simulink model "ModelWithSimulator"  (R2018a)
settings: Solver=ode4  StartTime=0.0  StopTime=inf  FixedStep=.001  RelTol=1e-2
undefined symbols (not defined in the file): car, initBeta, initR, initV
libraries: ephysenetlib x5, realtime_pacer_lib x1
settings Model: Creator=efrem  LastModifiedBy=efrem
settings SolverCC: AlgebraicLoopSolver=LineSearch
settings CodeAppCC: StateflowObjectComments=on

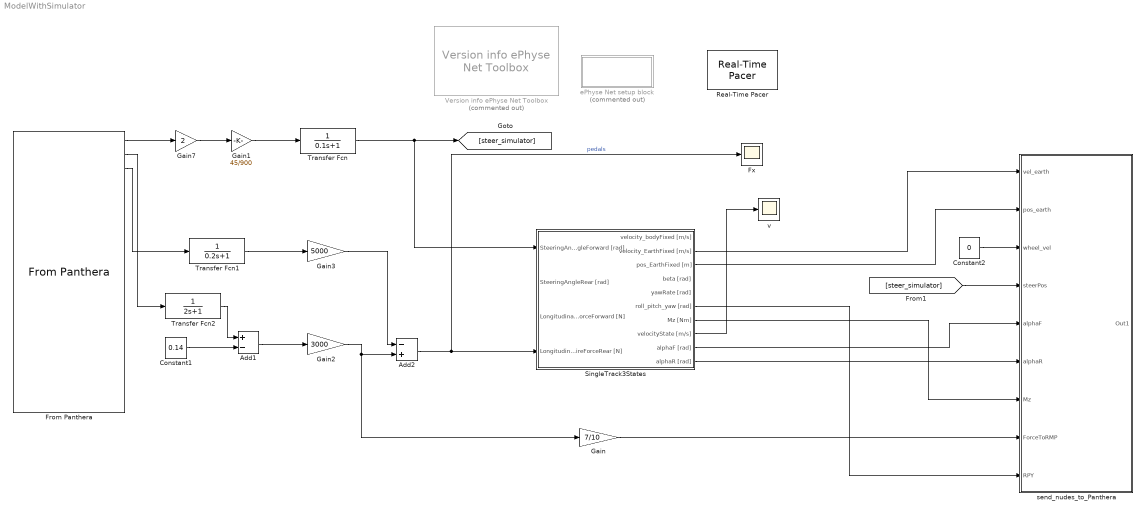
== system ModelWithSimulator ==
  Add1 : Sum  Inputs=+-
  Add2 : Sum  Inputs=-+
  Constant1 : Constant  Value=0.14
  Constant2 : Constant  Value=0
  From Panthera : ephysenetlib/Input blocks/From Panthera
  Fx : Scope
  Gain : Gain  Gain=7/10
  Gain1 : Gain  Gain=45/900
  Gain2 : Gain  Gain=3000
  Gain3 : Gain  Gain=5000
  Gain7 : Gain  Gain=2
  Real-Time Pacer : realtime_pacer_lib/Real-Time Pacer  simTimePerRealTime=1
  SingleTrack3States : Subsystem
  Transfer Fcn : TransferFcn  Denominator=[0.1 1]
  Transfer Fcn1 : TransferFcn  Denominator=[0.2 1]
  Transfer Fcn2 : TransferFcn  Denominator=[2 1]
  Version info ePhyse Net Toolbox : ephysenetlib/Setup blocks/Version info ePhyse Net Toolbox  Commented=on  InitialBlockCM=None  BlockCM=None  Frame=on  DisplayStringWithTags=|  HorizontalTextAlignment=Center  LeftAlignmentValue=0.5  SourceBlockDiagram=MODEL  TagMaxNumber=20
      | ePhyse Net Toolbox
      | Version:  1.0
      | Revision: $Rev: 1.0 $
      | 
      | © Cruden B.V., 2012
  ePhyse Net setup block : Subsystem  Commented=on  AncestorBlock=ephysenetlib/Setup blocks/Setup block
  send_nudes_to_Panthera : Subsystem
  v : Scope
  wires:
  SingleTrack3States/2(velocity_EarthFixed [m/s]) -> send_nudes_to_Panthera/1(vel_earth)
  Gain7/1 -> Gain1/1
  Gain1/1 -> Transfer Fcn/1
  SingleTrack3States/10(alphaR [rad]) -> send_nudes_to_Panthera/6(alphaR)
  Constant2/1 -> send_nudes_to_Panthera/3(wheel_vel)
  Constant1/1 -> Add1/2
  Transfer Fcn2/1 -> Add1/1
  Transfer Fcn1/1 -> Gain3/1
  From Panthera/2 -> Transfer Fcn2/1
  Add1/1 -> Gain2/1
  SingleTrack3States/9(alphaF [rad]) -> send_nudes_to_Panthera/5(alphaF)
  Add2/1 -> Fx/1, SingleTrack3States/4(LongitudinalTireForceRear [N])  "pedals"
  From Panthera/3 -> Transfer Fcn1/1
  SingleTrack3States/7(Mz [Nm]) -> send_nudes_to_Panthera/7(Mz)
  Gain2/1 -> Gain/1, Add2/2
  SingleTrack3States/3(pos_EarthFixed [m]) -> send_nudes_to_Panthera/2(pos_earth)
  Gain3/1 -> Add2/1
  SingleTrack3States/6(roll_pitch_yaw [rad]) -> send_nudes_to_Panthera/9("RPY ")
  [steer_simulator] -> send_nudes_to_Panthera/4(steerPos)
  From Panthera/1 -> Gain7/1
  Transfer Fcn/1 -> [steer_simulator], SingleTrack3States/1(SteeringAngleForward [rad])
  Gain/1 -> send_nudes_to_Panthera/8(ForceToRMP)
  SingleTrack3States/8(velocityState [m/s]) -> v/1

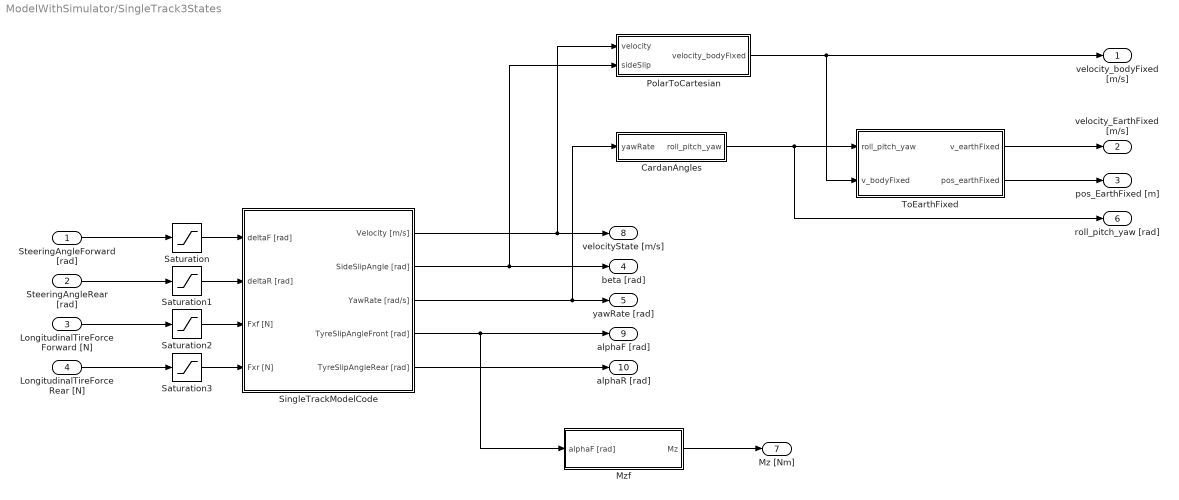
== system ModelWithSimulator/SingleTrack3States ==
  SteeringAngleForward [rad] : Inport
  SteeringAngleRear [rad] : Inport  Port=2
  LongitudinalTireForceForward [N] : Inport  Port=3
  LongitudinalTireForceRear [N] : Inport  Port=4
  CardanAngles : Subsystem
  Mzf : Subsystem
  PolarToCartesian : Subsystem
  Saturation : Saturate  UpperLimit=pi/3  LowerLimit=-pi/3  ZeroCross=off
  Saturation1 : Saturate  UpperLimit=pi/3  LowerLimit=-pi/3  ZeroCross=off
  Saturation2 : Saturate  UpperLimit=10000  LowerLimit=-10000  ZeroCross=off
  Saturation3 : Saturate  UpperLimit=10000  LowerLimit=-10000  ZeroCross=off
  SingleTrackModelCode : Subsystem
  ToEarthFixed : Subsystem
  velocity_bodyFixed [m/s] : Outport
  velocity_EarthFixed [m/s] : Outport  Port=2
  pos_EarthFixed [m] : Outport  Port=3
  beta [rad] : Outport  Port=4
  yawRate [rad] : Outport  Port=5
  roll_pitch_yaw [rad] : Outport  Port=6
  Mz [Nm] : Outport  Port=7
  velocityState [m/s] : Outport  Port=8
  alphaF [rad] : Outport  Port=9
  alphaR [rad] : Outport  Port=10
  wires:
  SingleTrackModelCode/3(YawRate [rad/s]) -> CardanAngles/1(yawRate), yawRate [rad]/1
  ToEarthFixed/2(pos_earthFixed) -> pos_EarthFixed [m]/1
  PolarToCartesian/1(velocity_bodyFixed) -> ToEarthFixed/2(v_bodyFixed), velocity_bodyFixed [m/s]/1
  SingleTrackModelCode/2(SideSlipAngle [rad]) -> PolarToCartesian/2(sideSlip), beta [rad]/1
  ToEarthFixed/1(v_earthFixed) -> velocity_EarthFixed [m/s]/1
  CardanAngles/1(roll_pitch_yaw) -> roll_pitch_yaw [rad]/1, ToEarthFixed/1(roll_pitch_yaw)
  SteeringAngleForward [rad]/1 -> Saturation/1
  LongitudinalTireForceForward [N]/1 -> Saturation2/1
  LongitudinalTireForceRear [N]/1 -> Saturation3/1
  Saturation1/1 -> SingleTrackModelCode/2(deltaR [rad])
  Saturation2/1 -> SingleTrackModelCode/3(Fxf [N])
  Saturation3/1 -> SingleTrackModelCode/4(Fxr [N])
  SteeringAngleRear [rad]/1 -> Saturation1/1
  Saturation/1 -> SingleTrackModelCode/1(deltaF [rad])
  SingleTrackModelCode/1(Velocity [m/s]) -> PolarToCartesian/1(velocity), velocityState [m/s]/1
  SingleTrackModelCode/4(TyreSlipAngleFront [rad]) -> Mzf/1(alphaF [rad]), alphaF [rad]/1
  SingleTrackModelCode/5(TyreSlipAngleRear [rad]) -> alphaR [rad]/1
  Mzf/1(Mz) -> Mz [Nm]/1

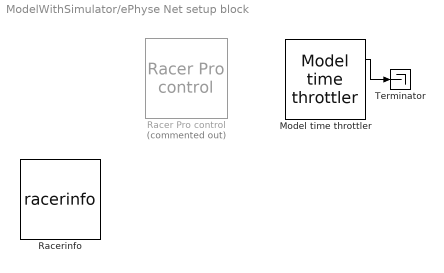
== system ModelWithSimulator/ePhyse Net setup block ==
  Model time throttler : ephysenetlib/Setup blocks/Model time throttler  enable=on
  Racer Pro control : ephysenetlib/Setup blocks/Racer Pro control  Commented=on
  Racerinfo : S-Function  Priority=5  FunctionName=racerinfo  Parameters=3  SFunctionDeploymentMode=off  EnableBusSupport=off
  Terminator : Terminator
  wires:
  Model time throttler/1 -> Terminator/1

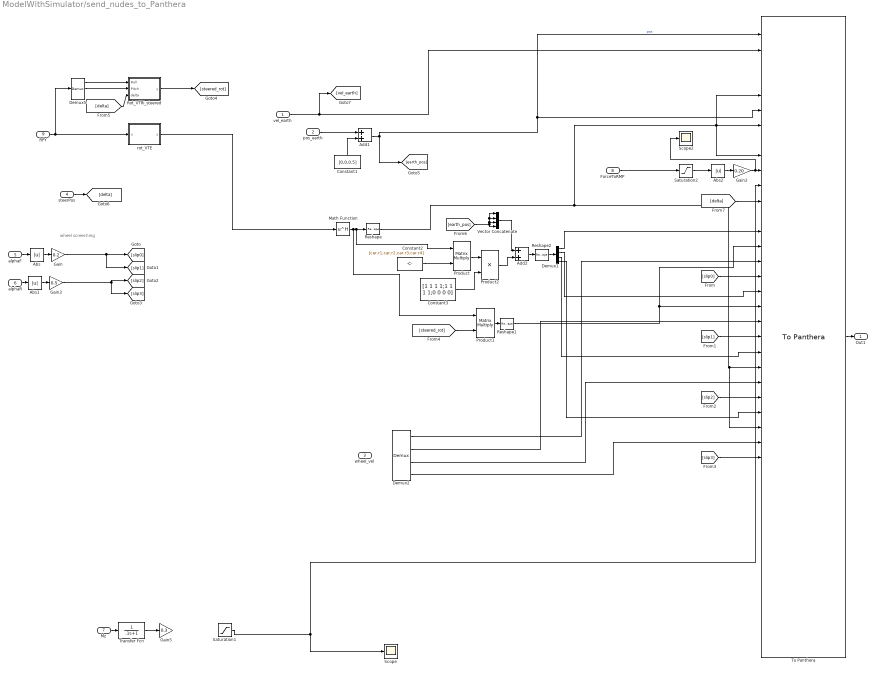
== system ModelWithSimulator/send_nudes_to_Panthera ==
  note: wheel screeching
  vel_earth : Inport
  pos_earth : Inport  Port=2
  wheel_vel : Inport  Port=3
  steerPos : Inport  Port=4
  alphaF : Inport  Port=5
  alphaR : Inport  Port=6
  Mz : Inport  Port=7
  ForceToRMP : Inport  Port=8
  "RPY " : Inport  Port=9
  Abs : Abs  ZeroCross=off
  Abs1 : Abs  ZeroCross=off
  Abs2 : Abs
  Add1 : Sum
  Add2 : Sum
  Constant1 : Constant  Value=[0,0,0.5]
  Constant2 : Constant  Value=[car.r1,car.r2,car.r3,car.r4]
  Constant3 : Constant  Value=[1 1 1 1;1 1 1 1;0 0 0 0]
  Demux1 : Demux
  Demux2 : Demux
  Demux5 : Demux  Outputs=3
  Gain : Gain  Gain=0.2
  Gain2 : Gain  Gain=0.20
  Gain3 : Gain  Gain=0.5
  Gain5 : Gain  Gain=0.3
  Math Function : Math  Operator=hermitian  SaturateOnIntegerOverflow=on
  Product : Product  Multiplication=Matrix(*)
  Product1 : Product  Multiplication=Matrix(*)
  Product2 : Product
  Reshape : Reshape
  Reshape1 : Reshape
  Reshape2 : Reshape  OutputDimensionality=Customize  OutputDimensions=[1,12]
  Rot_VTRi_steered : MATLAB Function  TreatAsAtomicUnit=on
  Saturation1 : Saturate  UpperLimit=150  LowerLimit=-150
  Saturation2 : Saturate  UpperLimit=inf  LowerLimit=0
  Scope : Scope
  Scope2 : Scope
  To Panthera : ephysenetlib/Output blocks/To Panthera
  Transfer Fcn : TransferFcn  Denominator=[.1 1]
  Vector Concatenate : Concatenate  NumInputs=4  Mode=Multidimensional array  ConcatenateDimension=2
  rot_VTE : MATLAB Function  TreatAsAtomicUnit=on
  Out1 : Outport
  wires:
  To Panthera/1 -> Out1/1
  vel_earth/1 -> [vel_earth], To Panthera/2
  rot_VTE/1(y) -> Math Function/1
  Math Function/1 -> Product1/1, Product/1, Reshape/1
  pos_earth/1 -> Add1/1
  Constant1/1 -> Add1/2
  [slip0] -> To Panthera/17
  [slip1] -> To Panthera/21
  [slip2] -> To Panthera/25
  [slip3] -> To Panthera/29
  Rot_VTRi_steered/1(y) -> [steered_rot]
  Constant2/1 -> Product/2
  Vector Concatenate/1 -> Add2/1
  [earth_pos] -> Vector Concatenate/4, Vector Concatenate/1, Vector Concatenate/2, Vector Concatenate/3
  Add2/1 -> Reshape2/1
  Reshape2/1 -> Demux1/1
  Demux1/1 -> To Panthera/14
  Demux1/2 -> To Panthera/18
  Demux1/3 -> To Panthera/22
  Demux1/4 -> To Panthera/26
  [steered_rot] -> Product1/2
  Product1/1 -> Reshape1/1
  Reshape1/1 -> To Panthera/15, To Panthera/19
  Reshape/1 -> To Panthera/9, To Panthera/5, To Panthera/7, To Panthera/27, To Panthera/23
  Add1/1 -> [earth_pos], To Panthera/6, To Panthera/1  "pos"
  Product/1 -> Product2/1
  Product2/1 -> Add2/2
  Constant3/1 -> Product2/2
  Demux2/1 -> To Panthera/16
  Demux2/2 -> To Panthera/20
  Demux2/3 -> To Panthera/24
  Demux2/4 -> To Panthera/28
  steerPos/1 -> [delta]
  alphaF/1 -> Abs/1
  Abs/1 -> Gain/1
  ForceToRMP/1 -> Saturation2/1
  Gain2/1 -> Scope2/1, To Panthera/10
  Abs2/1 -> Gain2/1
  Saturation2/1 -> Abs2/1
  "RPY "/1 -> rot_VTE/1(u), Demux5/1
  Demux5/1 -> Rot_VTRi_steered/1(Roll)
  Demux5/2 -> Rot_VTRi_steered/2(Pitch)
  [delta] -> Rot_VTRi_steered/3(delta)
  [delta] -> To Panthera/12
  Mz/1 -> Transfer Fcn/1
  Saturation1/1 -> To Panthera/11, Scope/1
  Abs1/1 -> Gain3/1
  alphaR/1 -> Abs1/1
  Gain/1 -> [slip1], [slip0]
  Gain3/1 -> [slip2], [slip3]
  Transfer Fcn/1 -> Gain5/1

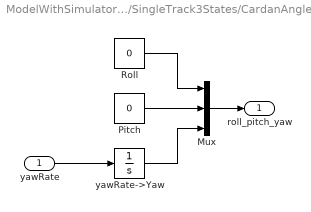
== system ModelWithSimulator/SingleTrack3States/CardanAngles ==
  yawRate : Inport
  Mux : Mux  Inputs=3
  Pitch : Constant  Value=0
  Roll : Constant  Value=0
  yawRate->Yaw : Integrator
  roll_pitch_yaw : Outport
  wires:
  Roll/1 -> Mux/1
  Mux/1 -> roll_pitch_yaw/1
  Pitch/1 -> Mux/2
  yawRate->Yaw/1 -> Mux/3
  yawRate/1 -> yawRate->Yaw/1

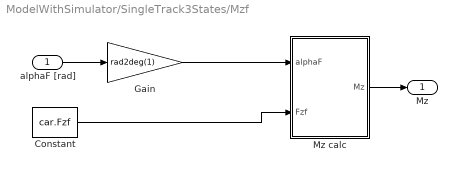
== system ModelWithSimulator/SingleTrack3States/Mzf ==
  alphaF [rad] : Inport
  Constant : Constant  Value=car.Fzf
  Gain : Gain  Gain=rad2deg(1)
  Mz calc : MATLAB Function  TreatAsAtomicUnit=on
  Mz : Outport
  wires:
  Mz calc/1(Mz) -> Mz/1
  Constant/1 -> Mz calc/2(Fzf)
  Gain/1 -> Mz calc/1(alphaF)
  alphaF [rad]/1 -> Gain/1

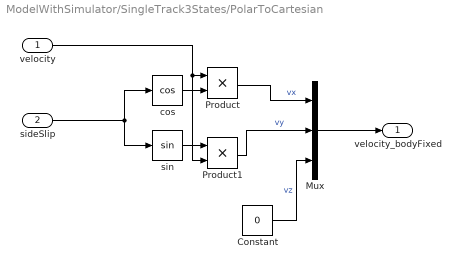
== system ModelWithSimulator/SingleTrack3States/PolarToCartesian ==
  velocity : Inport
  sideSlip : Inport  Port=2
  Constant : Constant  Value=0
  Mux : Mux  Inputs=3
  Product : Product
  Product1 : Product
  cos : Trigonometry  Operator=cos
  sin : Trigonometry
  velocity_bodyFixed : Outport
  wires:
  cos/1 -> Product/2
  sin/1 -> Product1/1
  Product/1 -> Mux/1  "vx"
  velocity/1 -> Product/1, Product1/2
  Product1/1 -> Mux/2  "vy"
  sideSlip/1 -> cos/1, sin/1
  Mux/1 -> velocity_bodyFixed/1
  Constant/1 -> Mux/3  "vz"

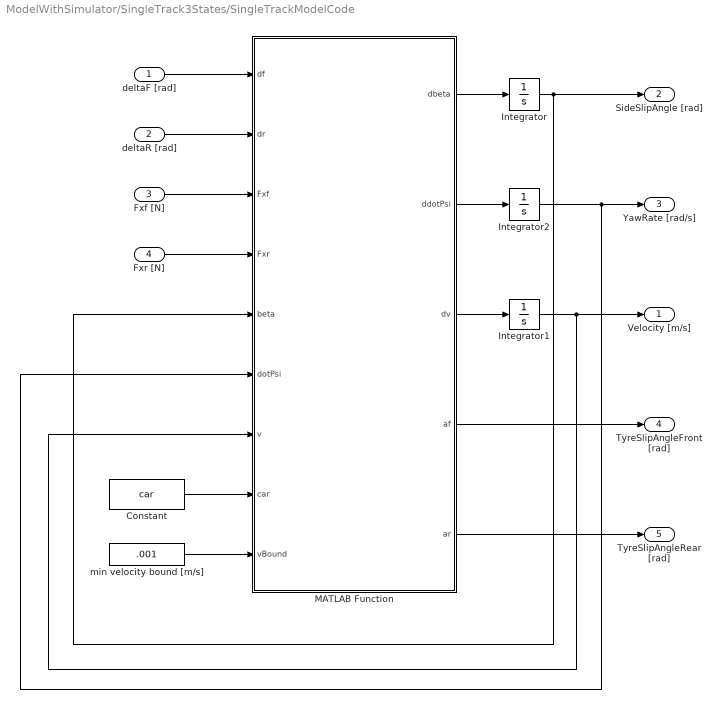
== system ModelWithSimulator/SingleTrack3States/SingleTrackModelCode ==
  deltaF [rad] : Inport
  deltaR [rad] : Inport  Port=2
  Fxf [N] : Inport  Port=3
  Fxr [N] : Inport  Port=4
  Constant : Constant  Value=car  OutDataTypeStr=Bus: car_bus
  Integrator : Integrator  InitialCondition=initBeta  UpperSaturationLimit=pi/2  LowerSaturationLimit=-pi/2  ZeroCross=off
  Integrator1 : Integrator  InitialCondition=initV  UpperSaturationLimit=100  LowerSaturationLimit=0.01  IgnoreLimit=on  ZeroCross=off
  Integrator2 : Integrator  InitialCondition=initR
  MATLAB Function : MATLAB Function  TreatAsAtomicUnit=on
  min velocity bound [m/s] : Constant  Value=.001
  Velocity [m/s] : Outport
  SideSlipAngle [rad] : Outport  Port=2
  YawRate [rad/s] : Outport  Port=3
  TyreSlipAngleFront [rad] : Outport  Port=4
  TyreSlipAngleRear [rad] : Outport  Port=5
  wires:
  MATLAB Function/1(dbeta) -> Integrator/1
  MATLAB Function/2(ddotPsi) -> Integrator2/1
  MATLAB Function/3(dv) -> Integrator1/1
  Integrator/1 -> SideSlipAngle [rad]/1, MATLAB Function/5(beta)
  Integrator2/1 -> YawRate [rad/s]/1, MATLAB Function/6(dotPsi)
  Integrator1/1 -> Velocity [m/s]/1, MATLAB Function/7(v)
  deltaF [rad]/1 -> MATLAB Function/1(df)
  deltaR [rad]/1 -> MATLAB Function/2(dr)
  Fxf [N]/1 -> MATLAB Function/3(Fxf)
  Fxr [N]/1 -> MATLAB Function/4(Fxr)
  min velocity bound [m/s]/1 -> MATLAB Function/9(vBound)
  MATLAB Function/4(af) -> TyreSlipAngleFront [rad]/1
  MATLAB Function/5(ar) -> TyreSlipAngleRear [rad]/1
  Constant/1 -> MATLAB Function/8(car)

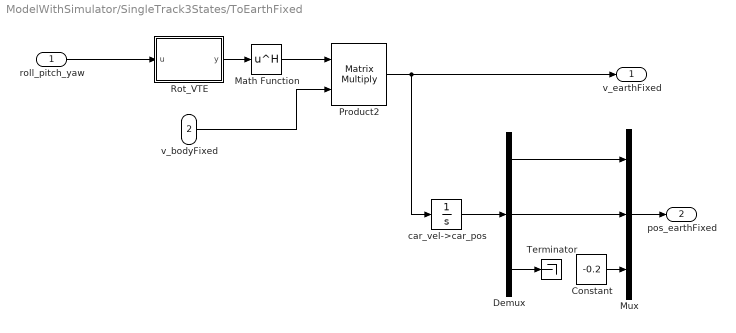
== system ModelWithSimulator/SingleTrack3States/ToEarthFixed ==
  roll_pitch_yaw : Inport
  v_bodyFixed : Inport  Port=2
  Constant : Constant  Value=-0.2
  Demux : Demux  Outputs=3
  Math Function : Math  Operator=hermitian  SaturateOnIntegerOverflow=on
  Mux : Mux  Inputs=3
  Product2 : Product  Multiplication=Matrix(*)
  Rot_VTE : MATLAB Function  TreatAsAtomicUnit=on
  Terminator : Terminator
  car_vel->car_pos : Integrator
  v_earthFixed : Outport
  pos_earthFixed : Outport  Port=2
  wires:
  Rot_VTE/1(y) -> Math Function/1
  roll_pitch_yaw/1 -> Rot_VTE/1(u)
  Constant/1 -> Mux/3
  car_vel->car_pos/1 -> Demux/1
  Product2/1 -> v_earthFixed/1, car_vel->car_pos/1
  Demux/1 -> Mux/1
  Demux/2 -> Mux/2
  v_bodyFixed/1 -> Product2/2
  Mux/1 -> pos_earthFixed/1
  Math Function/1 -> Product2/1
  Demux/3 -> Terminator/1

== matlab function ModelWithSimulator/SingleTrack3States/ToEarthFixed/Rot_VTE ==
  data: u input; y output
function y = fcn(u)
y = Rot_VTE(u);

== matlab function ModelWithSimulator/SingleTrack3States/Mzf/Mz calc ==
  data: alphaF input; Mz output; Fzf input
function Mz = fcn(alphaF, Fzf)
Bz = .15;
Cz = 2.3;
Dz = -.05 * Fzf;
Ez = -10;
Mz = Dz*sin((Cz*atan(Bz*alphaF - Ez*(Bz*alphaF - atan(Bz*alphaF)))));

== matlab function ModelWithSimulator/send_nudes_to_Panthera/rot_VTE ==
  data: u input; y output size=[3,3]
function y = fcn(u)
y = Rot_VTE(u);

== matlab function ModelWithSimulator/SingleTrack3States/SingleTrackModelCode/MATLAB Function ==
  data: df input; dbeta output; dr input; Fxf input; Fxr input; beta input; dotPsi input; v input; car input; vBound input; ddotPsi output; dv output; af output; ar output
function [dbeta, ddotPsi, dv, af, ar] = SingleTrackModelFunctionCode(df, dr, Fxf, Fxr, beta, dotPsi, v, car, vBound)
    
    %% parse parameters 
    lf = car.LF;
    lr = car.LR;
    m = car.Mass;
    Fzf = car.Fzf;
    Fzr = car.Fzb;
    Iz = car.Iz;
    D = car.Pacejka.D;
    B = car.Pacejka.B;
    C = car.Pacejka.C;
    E = car.Pacejka.E;

    %% deadzone for the velocity
    if(v < vBound && v >= 0) 
		v = v+vBound;
	elseif (v > -vBound && v <0)
        v = v-vBound;
    end
    
    %% kinematics
    af = -atan2((v*sin(beta)+lf*dotPsi)*cos(df)-v*cos(beta)*sin(df),...
        abs((v*sin(beta)+lf*dotPsi)*sin(df)+ v*cos(beta)*cos(df)));
    
    ar = -atan2((v*sin(beta)-lr*dotPsi)*cos(dr)-v*cos(beta)*sin(dr),...
        abs((v*sin(beta)-lr*dotPsi)*sin(dr)+ v*cos(beta)*cos(dr)));
    
    af_deg = rad2deg(af);
    ar_deg = rad2deg(ar);
    
    %% Pacejka 
    Fyf = D * Fzf * sin(C * atan(B*af_deg - E*(B*af_deg - atan(B*af_deg))));
    Fyr = D * Fzr * sin(C * atan(B*ar_deg - E*(B*ar_deg - atan(B*ar_deg))));

    %% steering angle projection and vehicle dynamics
    SAP = [cos(df), -sin(df), cos(dr), -sin(dr);...
        sin(df), cos(df), sin(dr), cos(dr);...
        lf*sin(df), lf*cos(df), -lr*sin(dr), -lr*cos(dr)];

    F = [Fxf; Fyf; Fxr; Fyr];

    RotDyn = [-sin(beta), cos(beta), 0;...
        cos(beta), sin(beta), 0;...
        0, 0, 1];

    Dyn = RotDyn * (SAP * F);
    
    % parse to motions
    lat = Dyn(1);
    long = Dyn(2);
    rot = Dyn(3);
	
    dbeta = - dotPsi + lat/m/v;
    dv = long/m;
    ddotPsi = rot/Iz;

end

== matlab function ModelWithSimulator/send_nudes_to_Panthera/Rot_VTRi_steered ==
  data: Roll input; y output; Pitch input; delta input
function y = fcn(Roll,Pitch,delta)
y = Rot_RiTV(Roll,Pitch,delta)';
